simulink model "lab06"  (R2023b)
settings: Solver=VariableStepAuto  StartTime=0.0  StopTime=10.0  RelTol=1e-3
libraries: spsDCVoltageSourceLib x2, spsDCMachineLib x1, sps_lib x1
settings Model: Creator=Shreetej  LastModifiedBy=Shreetej

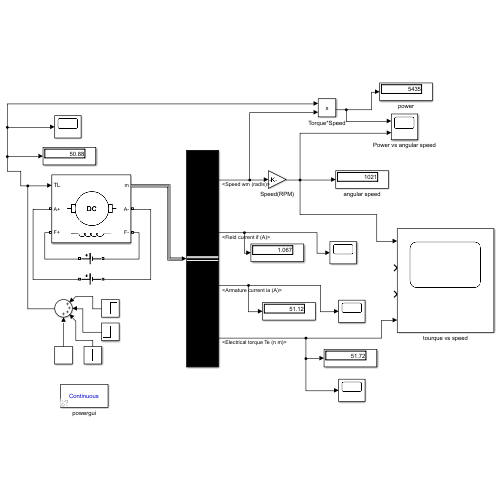
[thumbnail: Simulink's stored preview of the top-level diagram]
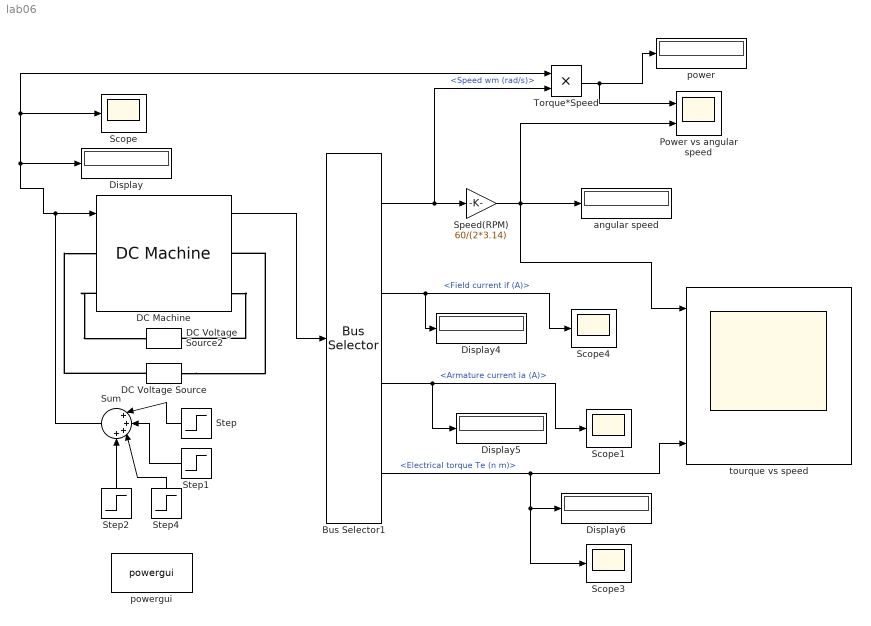
== system lab06 ==
  Bus Selector1 : BusSelector  OutputSignals=Speed wm (rad/s),Field current if (A),Armature current ia (A),Electrical torque Te (n m)
  DC Machine : spsDCMachineLib/DC Machine  PresetModel=01: 5HP 240V 1750RPM Field:300V  MechanicalLoad=Torque TL  FieldType=Wound  ShowDetailedParameters=on  MeasurementBus=off  RLa=[2.581 0.028]  RLf=[281.2 156]  Laf=0.9483  MachineConstant=Torque constant (N.m/A)  Ke=1.8  Kt=1.8  J=0.02215  Bm=0.002953  Tf=0.5161  w0=1  Ifinit=1.06685633001422  TsPowergui=0  TsBlock=-1
  DC Voltage Source : spsDCVoltageSourceLib/DC Voltage Source  Amplitude=240  Measurements=None
  DC Voltage Source2 : spsDCVoltageSourceLib/DC Voltage Source  Amplitude=300  Measurements=None
  Display{,4..6} (4 alike) : Display
  Power vs angular speed : Scope  NumInputPorts=2
  Scope{,1,3..4} (4 alike) : Scope
  Speed(RPM) : Gain  Gain=60/(2*3.14)
  Step : Step  Time=2  After=746*5*60/(2*pi*1750)*0.25  SampleTime=0
  Step1 : Step  Time=4  Before=746*5*60/(2*pi*1750)*0.25  After=746*5*60/(2*pi*1750)*0.5  SampleTime=0
  Step2 : Step  Time=8  Before=746*5*60/(2*pi*1750)*0.75  After=746*5*60/(2*pi*1750)  SampleTime=0
  Step4 : Step  Time=6  Before=746*5*60/(2*pi*1750)*0.5  After=746*5*60/(2*pi*1750)*0.75  SampleTime=0
  Sum : Sum  Inputs=|++++
  Torque*Speed : Product
  angular speed : Display
  power : Display
  powergui : sps_lib/powergui  Priority=1  SimulationMode=Continuous  SampleTime=50e-6  frequency=60  Iterations=50  frequencyindice=0  Pbase=100e6  ErrMax=1e-4  UnitsV=kV  UnitsW=MW  buscounter=0  FunctionMessages=off  echomessages=off  EnableUseOfTLC=off  CurrentSourceSwitches=off  DisableSnubberDevices=off  DisableRonSwitches=off  DisableVfSwitches=off  DisplayEquations=off  AutomaticDiscreteSolvers=off  SolverType=Tustin/Backward Euler (TBE)  Interpol=off  ExternalGateDelay=off  methode=off  Ts=100  x0status=blocks  SPID=on  SwTol=0  HookPort=off  NonlinearTolerance=1e-4  nMaxIteration=100  ContinueOnMaxIteration=off  RestoreLinks=warning  ResistiveCurrentMeasurement=off  Frange=[0:2:500]  Ylog=off  Xlog=on  ShowGrid=off  save=off  variable=ZData  structure=0  ZoomFFT=off  StartTime=0.0  cycles=1  DisplayStyle=1  fundamental=60  FreqAxis=off  MaxFrequency=1000  frequencyindicesteady=1  RmsSteady=1  display=off
  tourque vs speed : Scope  NumInputPorts=4
  wires:
  Sum/1 -> Torque*Speed/1, Scope/1, Display/1, DC Machine/1
  Step/1 -> Sum/1
  Step1/1 -> Sum/2
  Step4/1 -> Sum/3
  Torque*Speed/1 -> power/1, Power vs angular speed/1
  Step2/1 -> Sum/4
  DC Machine/1 -> Bus Selector1/1
  Bus Selector1/3 -> Scope1/1, Display5/1  "<Armature current ia (A)>"
  Bus Selector1/4 -> tourque vs speed/4, Scope3/1, Display6/1  "<Electrical torque Te (n m)>"
  Bus Selector1/1 -> Torque*Speed/2, Speed(RPM)/1  "<Speed wm (rad/s)>"
  Bus Selector1/2 -> Display4/1, Scope4/1  "<Field current if (A)>"
  Speed(RPM)/1 -> tourque vs speed/1, angular speed/1, Power vs angular speed/2
  connections:
  DC Voltage Source/RConn1 -- DC Machine/LConn1
  DC Voltage Source/LConn1 -- DC Machine/RConn1
  DC Machine/LConn2 -- DC Voltage Source2/RConn1
  DC Machine/RConn2 -- DC Voltage Source2/LConn1
